simulink model "DriveCycle_e8_IPMSM_HWJandVent_ROM"  (R2021b)
settings: Solver=VariableStepAuto  StartTime=0.0  StopTime=2474  FixedStep=1e-2  RelTol=1e-3  AbsTol=1e-3
model workspace (MAT data in the model file):
  AdjacencyMat = [0 0 0 0 0 0 0 0 0 0 0 0 ... (15129 elements, 123x123)]
  CapMat = [1e+20; 2196.70091586; 387.653102799; 193.8265514; 1962.34710525; 387.653102799; 193.8265514; 1962.34710525; 1266.59353814; 268.053957132; 416.539515956; 175.715078; 577.243160678; 310.101557898; 23.9530731873; 15.4990473565; 47.9061463746; 30.998094713; 85.98384; 1.11955442905; 1.11955442905; 1.11955442905; 1.11955442905; 1.11955442905; 1.11955442905; 0.373184809682; 0.373184809682; 450.202206395; 54.9511679003; 54.9511679003; 247.389926005; 247.389926005; 75.306462; 75.306462; 1.11955442905; 1.11955442905; 1e+20; 1e+20; 0; 0; 0; 0; 429.469897824; 0; 0; 0; 0; 429.469897824; 0; 0; 0; 0; 0; 0; 424.408023296; 268.053957132; 0; 0; 0; 0; 0; 322.102423368; 0; 0; 0; 0; 0; 322.102423368; 0; 0; 0; 0; 0; 318.306017472; 268.053957132; 2196.70091586; 1266.59353814; 268.053957132; 416.539515956; 175.715078; 577.243160678; 310.101557898; 85.98384; 0.373184809682; 0.373184809682; 450.202206395; 0; 0; 0; 0; 0; 424.408023296; 268.053957132; 0; 0; 0; 0; 318.306017472; 268.053957132; 2196.70091586; 1266.59353814; 268.053957132; 416.539515956; 175.715078; 577.243160678; 310.101557898; 85.98384; 0.373184809682; 0.373184809682; 450.202206395; 0; 0; 0; 0; 0; 424.408023296; 268.053957132; 0; 0; 0; 0; 318.306017472; 268.053957132]
  CoolantArrayIdxs = [20; 21; 22; 23; 24; 25; 26; 27; 35; 36; 37; 84; 85; 108; 109; 19; 38; 83; 107]
  Friction_Loss_Mat = [0 0 0 0 0 0 0 0 0 0 0 0 ... (2340 elements, 39x60)]
  InletCoolIdxs = [37; 38]
  Iron_Loss_Rotor_Back_Iron_Mat = [0.0117705351991 0.0198175800092 0.0246057415963 0.0256631766661 0.0240576767285 0.0207771722396 0.0168311502834 0.0133395315761 0.0115512535049 0.0120779527774 0.0143067244388 0.0171516443454 ... (2340 elements, 39x60)]
  Iron_Loss_Rotor_Pole_Mat = [1.45649756865 1.4525095653 1.42942652973 1.39109338754 1.34251579982 1.287439524 1.22885659237 1.16930852698 1.11098912611 1.05484046499 0.999976047808 0.944563732162 ... (2340 elements, 39x60)]
  Iron_Loss_Rotor_Tooth_Mat = [0 0 0 0 0 0 0 0 0 0 0 0 ... (2340 elements, 39x60)]
  Iron_Loss_Stator_Back_Iron_Mat = [38.5419456951 37.774471759 36.7837540443 35.6885758764 34.5272571596 33.3324529178 32.136302555 30.9744032473 29.8863152048 28.8790573391 27.8876077961 26.8074662049 ... (2340 elements, 39x60)]
  Iron_Loss_Stator_Tooth_Mat = [42.0610884508 41.0604961882 40.1804594162 39.4285940164 38.704339026 37.9602455604 37.1844153901 36.3902226975 35.6050856075 34.8287218867 34.0007237809 33.0439458619 ... (2340 elements, 39x60)]
  LossDistrForEachType = [0 0 0 0 0 0 0 0 0 0 0 0 ... (1968 elements, 16x123)]
  Magnet_Loss_Mat = [0.0995193918038 0.0928899922278 0.0868628846748 0.0818830115456 0.0774722500184 0.0732395922727 0.0687988836096 0.0636930921801 0.0573503948699 0.0496000064543 0.0410757743485 0.0326817704515 ... (2340 elements, 39x60)]
  OutletCoolIdxs = [20; 107]
  ResMat = [0 2.49009256841 6.64572241429 1000000000 1.39790968864 6.64402802995 1000000000 1.39156082742 1000000000 1000000000 1000000000 1000000000 ... (15129 elements, 123x123)]
  RotorCopperTempCoefResistivity = 0.00393
  Rotor_Cage_Loss_Mat = [0 0 0 0 0 0 0 0 0 0 0 0 ... (2340 elements, 39x60)]
  ShaftTorqueVec = [-287.262157301 -272.268610731 -257.275064161 -242.281517591 -227.287971021 -212.294424451 -197.300877881 -182.307331311 -167.31378474 -152.32023817 -137.3266916 -122.33314503 -107.33959846 -92.34605189 -77.35250532 -62.3589587499 -47.3654121798 -32.3718656097 -17.3783190396 -2.38477246955 12.6087741005 27.6023206706 42.5958672407 57.5894138108 72.5829603809 87.576506951 102.570053521 117.563600091 132.557146661 147.550693231 162.544239801 177.537786371 192.531332942 207.524879512 222.518426082 237.511972652 252.505519222 267.499065792 282.492612362]
  Sig = Simulink.Signal
  Sig.DataType = 'auto'
  Sig.Dimensions = -1
  Sig.DimensionsMode = 'auto'
  Sig.Complexity = 'auto'
  Sig.SampleTime = -1
  Sig.SamplingMode = 'auto'
  SpeedVec = [500 661.016949153 822.033898305 983.050847458 1144.06779661 1305.08474576 1466.10169492 1627.11864407 1788.13559322 1949.15254237 2110.16949153 2271.18644068 2432.20338983 2593.22033898 2754.23728814 2915.25423729 3076.27118644 3237.28813559 3398.30508475 3559.3220339 3720.33898305 3881.3559322 4042.37288136 4203.38983051 4364.40677966 4525.42372881 4686.44067797 4847.45762712 5008.47457627 5169.49152542 5330.50847458 5491.52542373 5652.54237288 5813.55932203 5974.57627119 6135.59322034 6296.61016949 6457.62711864 6618.6440678 6779.66101695 6940.6779661 7101.69491525 7262.71186441 7423.72881356 7584.74576271 7745.76271186 7906.77966102 8067.79661017 8228.81355932 8389.83050847 8550.84745763 8711.86440678 8872.88135593 9033.89830508 9194.91525424 9355.93220339 9516.94915254 9677.96610169 9838.98305085 10000]
  StateSpaceND : object (value not decoded)
  StatorCopperTempCoefResistivity = 0.00393
  Stator_Copper_Loss_Mat = [3925.33912093 3510.19452231 3089.33767218 2711.80000483 2370.99356953 2062.06508217 1781.35176729 1526.02799256 1293.87708125 1083.15658499 892.54525431 720.809889245 ... (2340 elements, 39x60)]
  Stray_Load_Loss_Mat = [0 0 0 0 0 0 0 0 0 0 0 0 ... (2340 elements, 39x60)]
  Stray_Loss_Stator_Iron_Proportion = 0.95
  Tgiven = 20
  TnodesInit = [25; 25; 25; 25; 25; 25; 25; 25; 25; 25; 25; 25; 25; 25; 25; 25; 25; 25; 25; 25; 25; 25; 25; 25; 25; 25; 25; 25; 25; 25; 25; 25; 25; 25; 25; 25; 25; 25; 25; 25; 25; 25; 25; 25; 25; 25; 25; 25; 25; 25; 25; 25; 25; 25; 25; 25; 25; 25; 25; 25; 25; 25; 25; 25; 25; 25; 25; 25; 25; 25; 25; 25; 25; 25; 25; 25; 25; 25; 25; 25; 25; 25; 25; 25; 25; 25; 25; 25; 25; 25; 25; 25; 25; 25; 25; 25; 25; 25; 25; 25; 25; 25; 25; 25; 25; 25; 25; 25; 25; 25; 25; 25; 25; 25; 25; 25; 25; 25; 25; 25; 25; 25; 25]
  TrefRotor = 20
  TrefStator = 20
  Windage_Loss_Mat = [0 0 0 0 0 0 0 0 0 0 0 0 ... (2340 elements, 39x60)]
libraries: mcadROM_lib x4, autolibshared x1, simulink x1
(part 1 of 2)
settings Model: Creator=agonzale  LastModifiedBy=agonzale
settings SolverCC: AutoScaleAbsTol=off

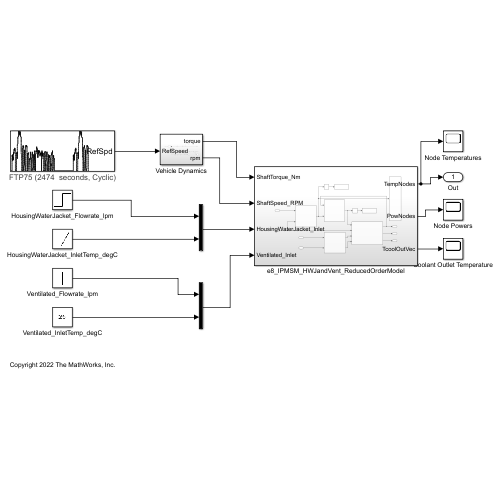
[thumbnail: Simulink's stored preview of the top-level diagram]
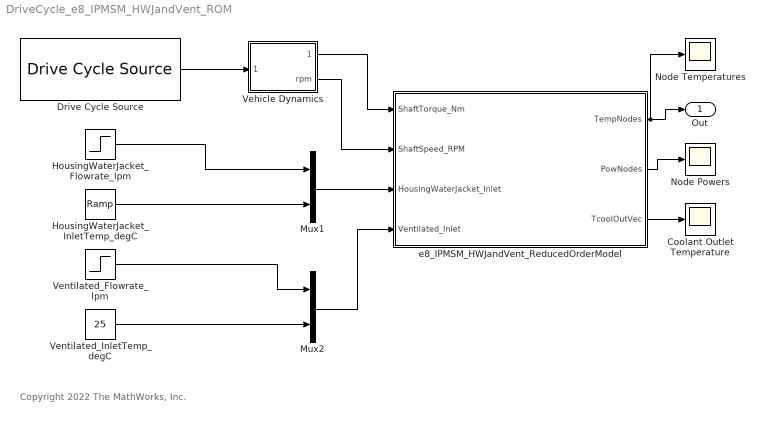
== system DriveCycle_e8_IPMSM_HWJandVent_ROM ==
  note: Copyright 2022 The MathWorks, Inc.
  Coolant Outlet Temperature : Scope
  Drive Cycle Source : autolibshared/Drive Cycle Source  cycleVar=FTP75  fileVar=cycleFTP75.mat  tfinal="2474  seconds, Cyclic"  cycleRepeat=on  outAccPort=off  outGearPort=off  gearList=No gear data  t_wot1=5  xdot_woto=0  xdot_wot1=30  t_wot2=20  xdot_wot2=0  t_wotend=30  srcUnit=m/s  outUnit=m/s  srcAccUnit=m/s/s  outAccUnit=m/s^2  dt=0  aMode=2  faultOption=off  velBnd=2  velBndUnit=mph  inUnit=m/s  timeBnd=1  failOption=off  stopSim=off  maxFaultCnt=10  maxFaultTime=2  maxTotFaultTime=15  traceOption=off  dtTrace=1  traceWindow=10  lastDCname=FTP75  lastOutUnit=mph  lastDT=0  lastTB=1  lastSB=2  forceCalcBound=off
      settings: SourceProductBaseCode=PW,DR,MT,UV,VE
  HousingWaterJacket_Flowrate_lpm : Step  Time=1000  Before=1  After=3  SampleTime=0
  HousingWaterJacket_InletTemp_degC : simulink/Sources/Ramp  slope=30/2474  start=0  InitialOutput=25
  Mux1 : Mux  Inputs=2
  Mux2 : Mux  Inputs=2
  Node Powers : Scope
  Node Temperatures : Scope
  Vehicle Dynamics : Subsystem
  Ventilated_Flowrate_lpm : Step  Time=1500  Before=2.5  After=7  SampleTime=0
  Ventilated_InletTemp_degC : Constant  Value=25
  e8_IPMSM_HWJandVent_ReducedOrderModel : Subsystem
  Out : Outport
  wires:
  e8_IPMSM_HWJandVent_ReducedOrderModel/2(PowNodes) -> Node Powers/1
  e8_IPMSM_HWJandVent_ReducedOrderModel/3(TcoolOutVec) -> Coolant Outlet Temperature/1
  HousingWaterJacket_Flowrate_lpm/1 -> Mux1/1
  Ventilated_Flowrate_lpm/1 -> Mux2/1
  Ventilated_InletTemp_degC/1 -> Mux2/2
  Mux2/1 -> e8_IPMSM_HWJandVent_ReducedOrderModel/4(Ventilated_Inlet)
  Mux1/1 -> e8_IPMSM_HWJandVent_ReducedOrderModel/3(HousingWaterJacket_Inlet)
  Vehicle Dynamics/2(rpm) -> e8_IPMSM_HWJandVent_ReducedOrderModel/2(ShaftSpeed_RPM)
  Vehicle Dynamics/1(torque) -> e8_IPMSM_HWJandVent_ReducedOrderModel/1(ShaftTorque_Nm)
  e8_IPMSM_HWJandVent_ReducedOrderModel/1(TempNodes) -> Node Temperatures/1, Out/1
  HousingWaterJacket_InletTemp_degC/1 -> Mux1/2
  Drive Cycle Source/1 -> Vehicle Dynamics/1(RefSpeed)
